simulink model "OrangeryTest"  (R2015a)
settings: configuration reference "GlobalConfig" (kept outside this file)
PreLoadFcn:
  | testModelPreLoadClbck
settings Model: CovSFcnEnable=off  Creator=Oleg_2  LastModifiedBy=Oleg
settings ConfigSetRef: SourceLocation=Base Workspace

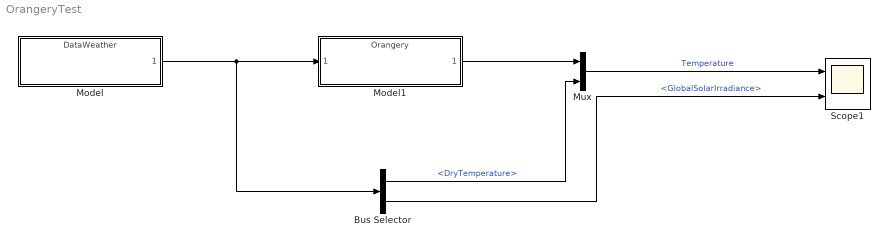
== system OrangeryTest ==
  Bus Selector : BusSelector  OutputSignals=DryTemperature,GlobalSolarIrradiance
  Model : ModelReference  ModelNameDialog=DataWeather.slx  SimulationMode=Normal  ModelReferenceVersion=1.65  CopyOfModelName=DataWeather.slx  DefaultDataLogging=on
  Model1 : ModelReference  ModelNameDialog=Orangery.slx  SimulationMode=Normal  ModelReferenceVersion=1.97  CopyOfModelName=Orangery.slx  DefaultDataLogging=on
  Mux : Mux  Inputs=2
  Scope1 : Scope  NumInputPorts=2
      settings: AttributesFormatString=%<AxesTitles>  TimeRange=169294.4312668461  YMin=273~0  YMax=294~1000  MaxDataPoints=1000000
  wires:
  Model/1 -> Model1/1, Bus Selector/1
  Model1/1 -> Mux/1
  Bus Selector/1 -> Mux/2  "<DryTemperature>"
  Mux/1 -> Scope1/1  "Temperature"
  Bus Selector/2 -> Scope1/2  "<GlobalSolarIrradiance>"
